simulink model "prach_shortFormat_fftShift_chanfix"  (R2022a)
settings: Solver=FixedStepDiscrete  StartTime=0.0  StopTime=prach_short.SimulationTime  FixedStep=1  RelTol=1e-3  EnableMultiTasking=on
PreLoadFcn:
  | warning off Simulink:Commands:SetParamLinkChangeWarn
  | warning off Simulink:Commands:LoadMdlParameterizedLink
  | warning off Simulink:SL_SetParamLinkChangeWarn
  | warning off Simulink:SL_LoadMdlParameterizedLink
  | setup_prach_shortFormat_fftShift;
InitFcn:
  | setup_prach_shortFormat_fftShift;
StopFcn:
  | figure;
  | subplot(3,1,1);
  | plot(real(X(:,1))/max(real(X(:,1))),'b');
  | hold on;
  | plot(imag(X(:,1))/max(real(X(:,1))),'r');
  | title('Raw FFT output, matlab reference');
  | subplot(3,1,2);
  | plot(real(PrachOut_DSPBA(1:Nfft))/max(real(PrachOut_DSPBA(1:Nfft))), 'k');
  | hold on;
  | plot(imag(PrachOut_DSPBA(1:Nfft))/max(imag(PrachOut_DSPBA(1:Nfft))), 'm');
  | title('Raw FFT output, DSP Builder');
  | subplot(3,1,3);
  | plot(real(X(:,1))/max(real(X(:,1)))-real(PrachOut_DSPBA(1:Nfft))/max(real(PrachOut_DSPBA(1:Nfft))), 'g');
  | hold on;
  | plot(imag(X(:,1))/max(real(X(:,1)))-imag(PrachOut_DSPBA(1:Nfft))/max(imag(PrachOut_DSPBA(1:Nfft))), 'c');
  | title('Difference');
  | 
  | figure;
  | subplot(2,1,1);
  | plot(real(prach_output(:,1))/max(real(prach_output(:,1))),'b');
  | hold on;
  | plot(imag(prach_output(:,1))/max(real(prach_output(:,1))),'r');
  | title('PRACH output, matlab, normalized ');
  | subplot(2,1,2);
  | for i=1:139
  |     PrachOut139reordered_DSPBA(1+PrachIdxOut139_DSPBA(i)) = PrachOut139_DSPBA(i);
  | end;
  | plot(real(PrachOut139reordered_DSPBA)/max(real(PrachOut139reordered_DSPBA)), 'k');
  | hold on;
  | plot(imag(PrachOut139reordered_DSPBA)/max(imag(PrachOut139reordered_DSPBA)), 'm');
  | title('PRACH output, DSP Builder, normalized');
values from neighbouring files (symbols this model uses):
  ConfigTable = [16 1 9,20,20,20,20,20,20,20,20,20 0 2 6 2 4 ... (first row only)    [ConfigIndexTable.m]
  NTxAnts = 4    [setup_prach_shortFormat.m]    (also in setup_prach_shortFormat_fftShift.m)
undefined symbols (not defined in the file or in its folder): AdvDSPBChannelOutDisplay, AdvDSPBDMemDisplay, BW, ControlDecode, display, dpoly, dspba, dspba_ChannelInVis, dspba_ChannelOutVis, dspba_internal_get_channel_ports, evalAionMaskParam, latency, PRACH_CC, PRACH_regs, prach_short, PrachLib, PrachLib_FFTshift, primtype, RemoveCP, Stream2BlockConv, UseDontCare, value, waveconfig
libraries: DSPBAPrim x326, DSPBAControl x10, DSPBAModelBus x7, DSPBABase x5, DSPBAUtilities x5, simulink x2, DSPBAVectorUtil x1, DspbAdvFftLibrary x1
(part 5 of 5)

== system prach_shortFormat_fftShift_chanfix/prach/PRACH_CC/Stream2BlockConv/WrCtrl/bitrev ==
  NatIn : Inport
  FFTSize : Inport  Port=2
  BitReverse : DSPBAPrim/BitReverse  primtype=bitrev  nInputs=1  nOutputs=1  omode=Inherit via internal rule  otype=sfix(16)  scale=2^-15  rndmethod=Unbiased  factor=1  satmethod=Symmetric  shift_vec=[0 1 2 -1]  value=0  inPortNames=[' '; ' ';]  outPortNames=[' ']  dspbaimage=dspba_prim.svg  text=fprintf('rev');  style=Optimised  visibilities=0  version=20211007
  Const2 : DSPBAPrim/Const  primtype=const  nInputs=0  nOutputs=1  omode=Inherit via internal rule  otype=sfix(16)  scale=2^-15  rndmethod=Unbiased  factor=1  satmethod=Symmetric  shift_vec=[0 1 2 -1]  value=log2(NFftMax)  inPortNames=['+'; '+';]  outPortNames=[' ']  dspbaimage=dspba_prim.svg  text=fprintf('%s', num2str(value));  style=Optimised  visibilities=8 + 1024  floatPrecision=float32_m23  warnSaturation=on  version=20211007  SampleTime=inf
  Shift : DSPBAPrim/Shift  primtype=shift  nInputs=2  nOutputs=1  omode=Specify via dialog  otype=ufix(ceil(log2(prach_short.Nfft)))  scale=1  rndmethod=Unbiased  factor=1  satmethod=Symmetric  shift_vec=[0 1 2 -1]  value=0  inPortNames=['a'; 'b';]  outPortNames=[' ']  dspbaimage=dspba_prim.svg  text=fprintf('a >> b');  style=Optimised  visibilities=8  version=20211007
  Sub : DSPBAPrim/Sub  primtype=sub  nInputs=2  nOutputs=1  omode=Specify via dialog  otype=ufix(4)  scale=1  rndmethod=Unbiased  factor=1  satmethod=Symmetric  shift_vec=[0 1 2 -1]  value=0  inPortNames=['+'; '-';]  outPortNames=[' ']  dspbaimage=dspba_prim.svg  text=fprintf('-');  style=Optimised  visibilities=8+2^17+2^18  floatRounding=correct  advOptions=[]  version=20211007
  WriteScope2 : Scope  NumInputPorts=4
  BitReversedOut : Outport
  NatOut : Outport  Port=2
  wires:
  BitReverse/1 -> WriteScope2/2, Shift/1
  NatIn/1 -> NatOut/1, WriteScope2/3, BitReverse/1
  FFTSize/1 -> Sub/2
  Const2/1 -> Sub/1
  Sub/1 -> Shift/2, WriteScope2/4
  Shift/1 -> WriteScope2/1, BitReversedOut/1
